simulink model "sy_tracking"  (R2020a)
settings: Solver=VariableStepAuto  StartTime=0.0  StopTime=50  FixedStep=0.001  MaxStep=0.001  RelTol=1e-3  EnableMultiTasking=on
values from neighbouring files (symbols this model uses):
  a11 = -70/3085    (= -0.0226904376013)    [sy_tracking_1.m]
  a12 = -2642.7/3085*u0    (= 0)    [sy_tracking_1.m]
  a21 = -442.2/915.5*u0    (= 0)    [sy_tracking_1.m]
  a22 = -105/915.5    (= -0.114691425451)    [sy_tracking_1.m]
  b1 = 1/3085    (= 0.00032414910859)    [sy_tracking_1.m]
  F = [K eye(mm)]*inv(TT)    [sy_tracking_1.m]
  N_r_bar = -523.27/915.5    (= -0.571567449481)    [sy_tracking_1.m]
  Y_v_bar = -992/3085    (= -0.321555915721)    [sy_tracking_1.m]
settings Model: Creator=xiaoran  LastModifiedBy=xiaoran
settings DataIOCC: LimitDataPoints=on  SaveFormat=Array  ReturnWorkspaceOutputs=off
settings OptimizationCC: LifeSpan=inf
settings DebuggingCC: UnderspecifiedInitializationDetection=Classic  MergeDetectMultiDrivingBlocksExec=none  SolverPrmCheckMsg=warning  StateNameClashWarn=warning  SFUnexpectedBacktrackingDiag=warning  SFNoUnconditionalDefaultTransitionDiag=warning  SFExecutionAtInitializationDiag=none  ArithmeticOperatorsInVariantConditions=warning
settings HardwareCC: ProdBitPerPointer=32  ProdBitPerSizeT=32  ProdBitPerPtrDiffT=32  ProdLargestAtomicFloat=None  ProdIntDivRoundTo=Undefined  ProdEndianess=Unspecified  ProdWordSize=32  ProdHWDeviceType=32-bit Generic
settings ModelReferenceCC: PropagateSignalLabelsOutOfModel=off
settings SFSimCC: SimUseLocalCustomCode=off  CustomCodeUndefinedFunction=UseInterfaceOnly
settings RTWCC: RTWUseLocalCustomCode=off
settings CodeAppCC: StateflowObjectComments=on
settings GRTTargetCC: TargetLangStandard=C89/C90 (ANSI)
settings ConfigComp: CovMetricSettings=dw  CovHtmlReporting=on  CovSaveCumulativeToWorkspaceVar=on  CovSaveSingleToWorkspaceVar=on  CovExternalEMLEnable=off

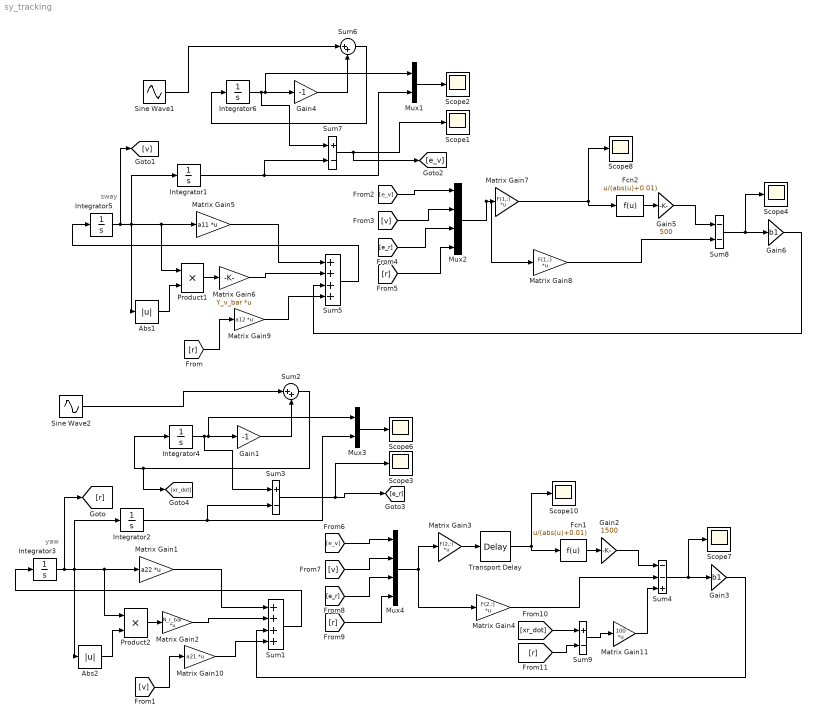
== system sy_tracking ==
  note: yaw
  note: sway
  Abs1 : Abs
  Abs2 : Abs
  Fcn1 : Fcn  Expr=u/(abs(u)+0.01)
  Fcn2 : Fcn  Expr=u/(abs(u)+0.01)
  Gain1 : Gain  Gain=-1
  Gain2 : Gain  Gain=1500  SaturateOnIntegerOverflow=on  OutDataTypeStr=Inherit: Same as input  ParamDataTypeStr=Inherit: Same as input
  Gain3 : Gain  Gain=b1  SaturateOnIntegerOverflow=on  OutDataTypeStr=Inherit: Same as input  ParamDataTypeStr=Inherit: Same as input
  Gain4 : Gain  Gain=-1
  Gain5 : Gain  Gain=500  SaturateOnIntegerOverflow=on  OutDataTypeStr=Inherit: Same as input  ParamDataTypeStr=Inherit: Same as input
  Gain6 : Gain  Gain=b1  SaturateOnIntegerOverflow=on  OutDataTypeStr=Inherit: Same as input  ParamDataTypeStr=Inherit: Same as input
  Integrator{1..3,5} (4 alike) : Integrator  InitialCondition=0.1
  Integrator4 : Integrator  InitialCondition=.1
  Integrator6 : Integrator  InitialCondition=.1
  Matrix Gain1 : Gain  Gain=a22  Multiplication=Matrix(K*u)  SaturateOnIntegerOverflow=on  OutDataTypeStr=Inherit: Same as input  ParamDataTypeStr=Inherit: Same as input
  Matrix Gain10 : Gain  Gain=a21  Multiplication=Matrix(K*u)  SaturateOnIntegerOverflow=on  OutDataTypeStr=Inherit: Same as input  ParamDataTypeStr=Inherit: Same as input
  Matrix Gain11 : Gain  Gain=100  Multiplication=Matrix(K*u)  SaturateOnIntegerOverflow=on  OutDataTypeStr=Inherit: Same as input  ParamDataTypeStr=Inherit: Same as input
  Matrix Gain2 : Gain  Gain=N_r_bar  Multiplication=Matrix(K*u)  SaturateOnIntegerOverflow=on  OutDataTypeStr=Inherit: Same as input  ParamDataTypeStr=Inherit: Same as input
  Matrix Gain3 : Gain  Gain=F(2,:)  Multiplication=Matrix(K*u)  SaturateOnIntegerOverflow=on  OutDataTypeStr=Inherit: Same as input  ParamDataTypeStr=Inherit: Same as input
  Matrix Gain4 : Gain  Gain=F(2,:)  Multiplication=Matrix(K*u)  SaturateOnIntegerOverflow=on  OutDataTypeStr=Inherit: Same as input  ParamDataTypeStr=Inherit: Same as input
  Matrix Gain5 : Gain  Gain=a11  Multiplication=Matrix(K*u)  SaturateOnIntegerOverflow=on  OutDataTypeStr=Inherit: Same as input  ParamDataTypeStr=Inherit: Same as input
  Matrix Gain6 : Gain  Gain=Y_v_bar  Multiplication=Matrix(K*u)  SaturateOnIntegerOverflow=on  OutDataTypeStr=Inherit: Same as input  ParamDataTypeStr=Inherit: Same as input
  Matrix Gain7 : Gain  Gain=F(1,:)  Multiplication=Matrix(K*u)  SaturateOnIntegerOverflow=on  OutDataTypeStr=Inherit: Same as input  ParamDataTypeStr=Inherit: Same as input
  Matrix Gain8 : Gain  Gain=F(1,:)  Multiplication=Matrix(K*u)  SaturateOnIntegerOverflow=on  OutDataTypeStr=Inherit: Same as input  ParamDataTypeStr=Inherit: Same as input
  Matrix Gain9 : Gain  Gain=a12  Multiplication=Matrix(K*u)  SaturateOnIntegerOverflow=on  OutDataTypeStr=Inherit: Same as input  ParamDataTypeStr=Inherit: Same as input
  Mux1 : Mux  Inputs=2
  Mux2 : Mux
  Mux3 : Mux  Inputs=2
  Mux4 : Mux
  Product1 : Product
  Product2 : Product
  Scope{1..4,6..8,10} (8 alike) : Scope
  Sine Wave1 : Sin  SampleTime=0
  Sine Wave2 : Sin  Amplitude=.5  SampleTime=0
  Sum1 : Sum  Inputs=++++  InputSameDT=on  SaturateOnIntegerOverflow=on  OutDataTypeStr=Inherit: Same as first input
  Sum2 : Sum  Inputs=|++
  Sum3 : Sum  Inputs=+-  InputSameDT=on  SaturateOnIntegerOverflow=on  OutDataTypeStr=Inherit: Same as first input
  Sum4 : Sum  Inputs=--+  InputSameDT=on  SaturateOnIntegerOverflow=on  OutDataTypeStr=Inherit: Same as first input
  Sum5 : Sum  Inputs=++++  InputSameDT=on  SaturateOnIntegerOverflow=on  OutDataTypeStr=Inherit: Same as first input
  Sum6 : Sum  Inputs=|++
  Sum7 : Sum  Inputs=+-  InputSameDT=on  SaturateOnIntegerOverflow=on  OutDataTypeStr=Inherit: Same as first input
  Sum8 : Sum  Inputs=--  InputSameDT=on  SaturateOnIntegerOverflow=on  OutDataTypeStr=Inherit: Same as first input
  Sum9 : Sum  Inputs=+-  InputSameDT=on  SaturateOnIntegerOverflow=on  OutDataTypeStr=Inherit: Same as first input
  Transport Delay : TransportDelay  DelayTime=0
  wires:
  Abs1/1 -> Product1/2
  Product1/1 -> Matrix Gain6/1
  Matrix Gain5/1 -> Sum5/1
  Matrix Gain6/1 -> Sum5/2
  Sum5/1 -> Integrator5/1
  Sum6/1 -> Integrator6/1
  Gain4/1 -> Sum6/2
  Integrator6/1 -> Mux1/1, Gain4/1, Sum7/1
  Integrator5/1 -> [v], Integrator1/1, Abs1/1, Product1/1, Matrix Gain5/1
  Sum7/1 -> [e_v], Scope1/1
  Mux2/1 -> Matrix Gain7/1, Matrix Gain8/1
  Fcn2/1 -> Gain5/1
  Sum8/1 -> Scope4/1, Gain6/1
  Gain6/1 -> Sum5/3
  Mux1/1 -> Scope2/1
  Sine Wave1/1 -> Sum6/1
  Integrator1/1 -> Mux1/2, Sum7/2
  Matrix Gain7/1 -> Fcn2/1, Scope8/1
  Gain5/1 -> Sum8/1
  Matrix Gain3/1 -> Transport Delay/1
  Integrator2/1 -> Sum3/2, Mux3/2
  Sine Wave2/1 -> Sum2/1
  Mux3/1 -> Scope6/1
  Gain3/1 -> Sum1/3
  Sum4/1 -> Gain3/1, Scope7/1
  Fcn1/1 -> Gain2/1
  Mux4/1 -> Matrix Gain3/1, Matrix Gain4/1
  Sum3/1 -> [e_r], Scope3/1
  Integrator3/1 -> [r], Matrix Gain1/1, Product2/1, Abs2/1, Integrator2/1
  Integrator4/1 -> Sum3/1, Gain1/1, Mux3/1
  Gain1/1 -> Sum2/2
  Sum2/1 -> [xr_dot], Integrator4/1
  Sum1/1 -> Integrator3/1
  Matrix Gain2/1 -> Sum1/2
  Matrix Gain1/1 -> Sum1/1
  Product2/1 -> Matrix Gain2/1
  Abs2/1 -> Product2/2
  [r] -> Matrix Gain9/1
  Matrix Gain9/1 -> Sum5/4
  [v] -> Matrix Gain10/1
  Matrix Gain10/1 -> Sum1/4
  [e_v] -> Mux2/1
  [v] -> Mux2/2
  [e_r] -> Mux2/3
  [r] -> Mux2/4
  [e_v] -> Mux4/1
  [v] -> Mux4/2
  [e_r] -> Mux4/3
  [r] -> Mux4/4
  Transport Delay/1 -> Scope10/1, Fcn1/1
  [xr_dot] -> Sum9/1
  [r] -> Sum9/2
  Sum9/1 -> Matrix Gain11/1
  Matrix Gain11/1 -> Sum4/3
  Gain2/1 -> Sum4/1
  Matrix Gain8/1 -> Sum8/2
  Matrix Gain4/1 -> Sum4/2
